simulink model "LowSpeed"  (R2022b)
settings: Solver=FixedStepDiscrete  StartTime=0.0  StopTime=10.0  FixedStep=0.0001  RelTol=1e-3
undefined symbols (not defined in the file or in its folder): DEPOWER_FLAG, DEPOWER_NO_FLAG, ParamCfg_IsMax_u16, ParamCfg_LowSpeedCoeff_u16, ParamCfg_LowSpeedDelay_u16, ParamCfg_LowSpeedGain_u16, ParamCfg_MaxTorque_u16, ParamCfg_SpeedLowLimit_u16
libraries: simulink x2
settings Model: DataDictionary=MCU_LowSpeed.sldd  Creator=ZYH  LastModifiedBy=ZYH
settings OptimizationCC: DefaultParameterBehavior=Inlined  EnhancedBackFolding=on  PassReuseOutputArgsAs=Individual arguments  ZeroExternalMemoryAtStartup=off  ZeroInternalMemoryAtStartup=off  OptimizeBlockOrder=speed  DifferentSizesBufferReuse=on  OptimizationCustomize=off  EfficientTunableParamExpr=on
settings DebuggingCC: ParameterTunabilityLossMsg=error
settings SFSimCC: MATLABDynamicMemAlloc=off
settings RTWCC: Description=Embedded Coder  SystemTargetFile=ert.tlc  GenCodeOnly=on  TemplateMakefile=ert_default_tmf
settings CodeAppCC: ForceParamTrailComments=on  IgnoreCustomStorageClasses=off  OperatorAnnotations=on  SimulinkDataObjDesc=on  SFDataObjDesc=on  InsertBlockDesc=on
settings ERTTargetCC: TargetLangStandard=C99 (ISO)  GenerateSampleERTMain=on  InlinedParameterPlacement=NonHierarchical  ERTCustomFileTemplate=example_file_process.tlc

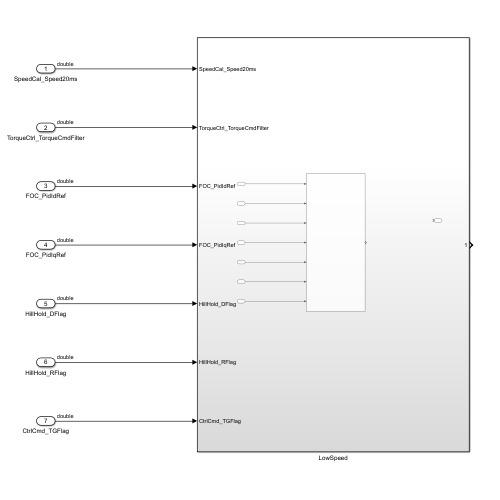
[thumbnail: Simulink's stored preview of the top-level diagram]
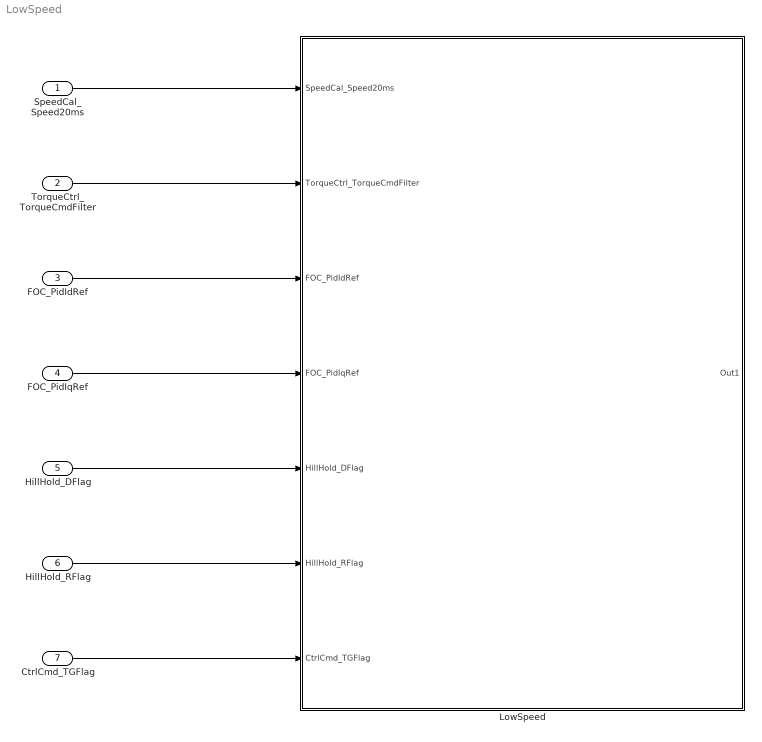
== system LowSpeed ==
  SpeedCal_Speed20ms : Inport
  TorqueCtrl_TorqueCmdFilter : Inport  Port=2
  FOC_PidIdRef : Inport  Port=3
  FOC_PidIqRef : Inport  Port=4
  HillHold_DFlag : Inport  Port=5
  HillHold_RFlag : Inport  Port=6
  CtrlCmd_TGFlag : Inport  Port=7
  LowSpeed : Subsystem
  wires:
  SpeedCal_Speed20ms/1 -> LowSpeed/1(SpeedCal_Speed20ms)
  TorqueCtrl_TorqueCmdFilter/1 -> LowSpeed/2(TorqueCtrl_TorqueCmdFilter)
  FOC_PidIdRef/1 -> LowSpeed/3(FOC_PidIdRef)
  FOC_PidIqRef/1 -> LowSpeed/4(FOC_PidIqRef)
  HillHold_DFlag/1 -> LowSpeed/5(HillHold_DFlag)
  HillHold_RFlag/1 -> LowSpeed/6(HillHold_RFlag)
  CtrlCmd_TGFlag/1 -> LowSpeed/7(CtrlCmd_TGFlag)

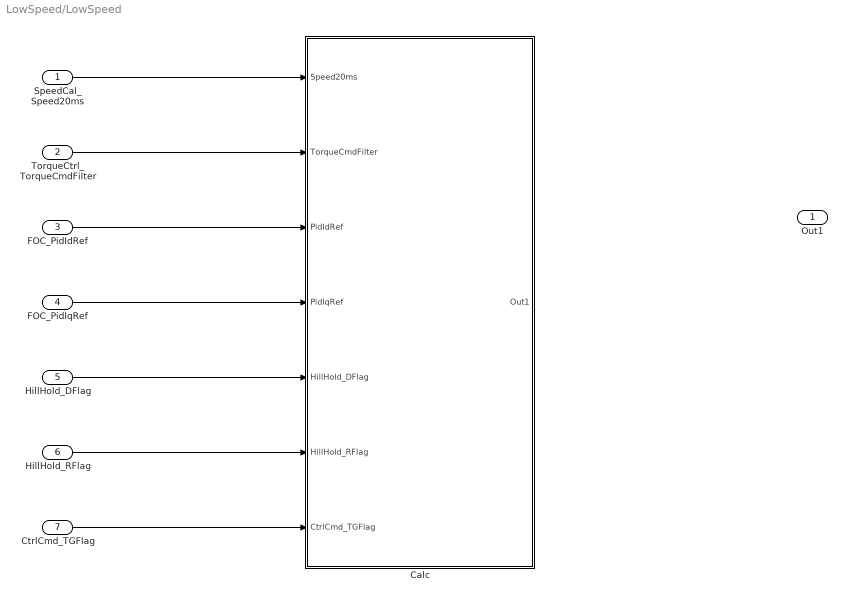
== system LowSpeed/LowSpeed ==
  SpeedCal_Speed20ms : Inport
  TorqueCtrl_TorqueCmdFilter : Inport  Port=2
  FOC_PidIdRef : Inport  Port=3
  FOC_PidIqRef : Inport  Port=4
  HillHold_DFlag : Inport  Port=5
  HillHold_RFlag : Inport  Port=6
  CtrlCmd_TGFlag : Inport  Port=7
  Calc : Subsystem
  Out1 : Outport
  wires:
  SpeedCal_Speed20ms/1 -> Calc/1(Speed20ms)
  TorqueCtrl_TorqueCmdFilter/1 -> Calc/2(TorqueCmdFilter)
  FOC_PidIdRef/1 -> Calc/3(PidIdRef)
  FOC_PidIqRef/1 -> Calc/4(PidIqRef)
  HillHold_DFlag/1 -> Calc/5(HillHold_DFlag)
  HillHold_RFlag/1 -> Calc/6(HillHold_RFlag)
  CtrlCmd_TGFlag/1 -> Calc/7(CtrlCmd_TGFlag)

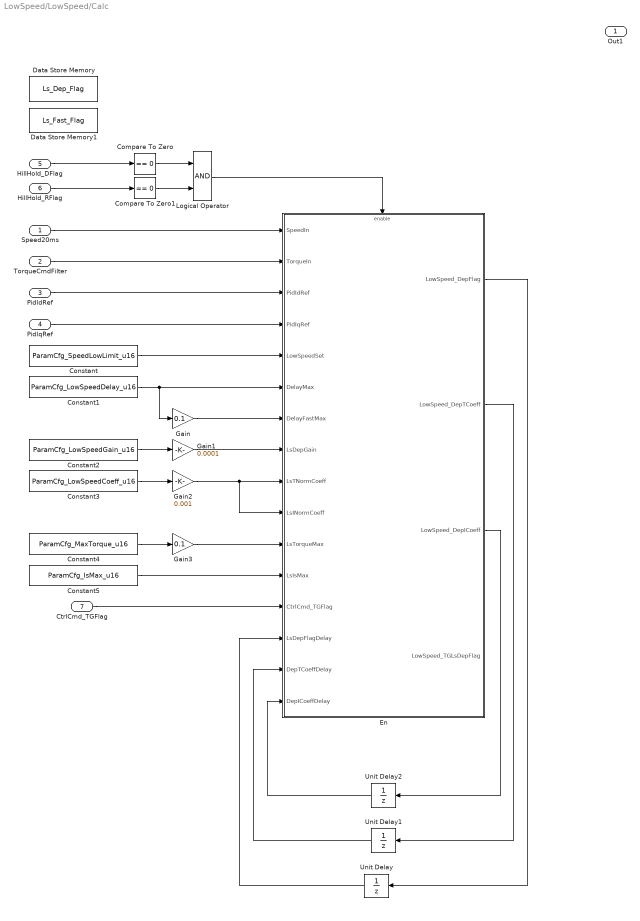
== system LowSpeed/LowSpeed/Calc ==
  Speed20ms : Inport
  TorqueCmdFilter : Inport  Port=2
  PidIdRef : Inport  Port=3
  PidIqRef : Inport  Port=4
  HillHold_DFlag : Inport  Port=5
  HillHold_RFlag : Inport  Port=6
  CtrlCmd_TGFlag : Inport  Port=7
  Compare To Zero : simulink/Logic and Bit Operations/Compare To Zero  relop===  OutDataTypeStr=boolean
  Compare To Zero1 : simulink/Logic and Bit Operations/Compare To Zero  relop===  OutDataTypeStr=boolean
  Constant : Constant  Value=ParamCfg_SpeedLowLimit_u16
  Constant1 : Constant  Value=ParamCfg_LowSpeedDelay_u16
  Constant2 : Constant  Value=ParamCfg_LowSpeedGain_u16
  Constant3 : Constant  Value=ParamCfg_LowSpeedCoeff_u16
  Constant4 : Constant  Value=ParamCfg_MaxTorque_u16
  Constant5 : Constant  Value=ParamCfg_IsMax_u16  VectorParams1D=off
  Data Store Memory : DataStoreMemory  DataStoreName=Ls_Dep_Flag  WriteAfterWriteMsg=warning  InitialValue=DEPOWER_NO_FLAG  ShowAdditionalParam=off  OutDataTypeStr=uint8
  Data Store Memory1 : DataStoreMemory  DataStoreName=Ls_Fast_Flag  WriteAfterWriteMsg=warning  InitialValue=false  ShowAdditionalParam=off  OutDataTypeStr=uint8
  En : Subsystem  TreatAsAtomicUnit=on
  Gain : Gain  Gain=0.1  ParamDataTypeStr=single  OutDataTypeStr=single
  Gain1 : Gain  Gain=0.0001  ParamDataTypeStr=single  OutDataTypeStr=single
  Gain2 : Gain  Gain=0.001  ParamDataTypeStr=single  OutDataTypeStr=single
  Gain3 : Gain  Gain=0.1  ParamDataTypeStr=single  OutDataTypeStr=single
  Logical Operator : Logic  AllPortsSameDT=off  OutDataTypeStr=boolean
  Unit Delay : UnitDelay  SampleTime=-1  HasFrameUpgradeWarning=on
  Unit Delay1 : UnitDelay  SampleTime=-1  HasFrameUpgradeWarning=on
  Unit Delay2 : UnitDelay  SampleTime=-1  HasFrameUpgradeWarning=on
  Out1 : Outport
  wires:
  HillHold_DFlag/1 -> Compare To Zero/1
  HillHold_RFlag/1 -> Compare To Zero1/1
  Compare To Zero1/1 -> Logical Operator/2
  Compare To Zero/1 -> Logical Operator/1
  Logical Operator/1 -> En/Enable
  Speed20ms/1 -> En/1(SpeedIn)
  TorqueCmdFilter/1 -> En/2(TorqueIn)
  PidIdRef/1 -> En/3(PidIdRef)
  PidIqRef/1 -> En/4(PidIqRef)
  Constant/1 -> En/5(LowSpeedSet)
  Gain/1 -> En/7(DelayFastMax)
  Constant1/1 -> Gain/1, En/6(DelayMax)
  Constant2/1 -> Gain1/1
  Gain1/1 -> En/8(LsDepGain)
  Constant3/1 -> Gain2/1
  Gain2/1 -> En/10(LsINormCoeff), En/9(LsTNormCoeff)
  Constant4/1 -> Gain3/1
  Gain3/1 -> En/11(LsTorqueMax)
  Constant5/1 -> En/12(LsIsMax)
  En/1(LowSpeed_DepFlag) -> Unit Delay/1
  Unit Delay/1 -> En/14(LsDepFlagDelay)
  En/2(LowSpeed_DepTCoeff) -> Unit Delay1/1
  Unit Delay1/1 -> En/15(DepTCoeffDelay)
  En/3(LowSpeed_DepICoeff) -> Unit Delay2/1
  Unit Delay2/1 -> En/16(DepICoeffDelay)
  CtrlCmd_TGFlag/1 -> En/13(CtrlCmd_TGFlag)

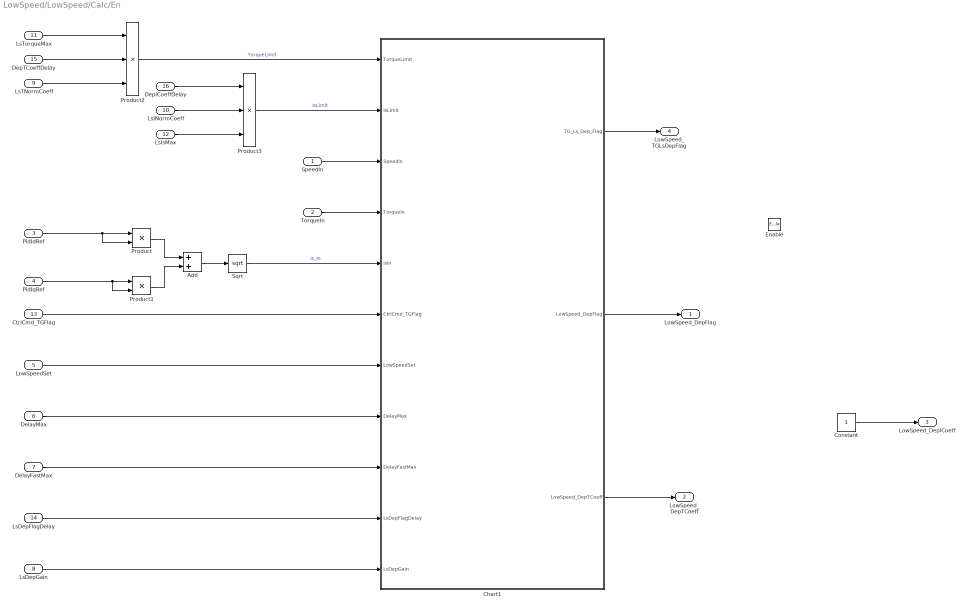
== system LowSpeed/LowSpeed/Calc/En ==
  SpeedIn : Inport
  TorqueIn : Inport  Port=2
  PidIdRef : Inport  Port=3
  PidIqRef : Inport  Port=4
  LowSpeedSet : Inport  Port=5
  DelayMax : Inport  Port=6
  DelayFastMax : Inport  Port=7
  LsDepGain : Inport  Port=8
  LsTNormCoeff : Inport  Port=9
  LsINormCoeff : Inport  Port=10
  LsTorqueMax : Inport  Port=11
  LsIsMax : Inport  Port=12
  CtrlCmd_TGFlag : Inport  Port=13
  LsDepFlagDelay : Inport  Port=14
  DepTCoeffDelay : Inport  Port=15
  DepICoeffDelay : Inport  Port=16
  Enable : EnablePort
  Add : Sum
  Chart1 : Stateflow chart  TreatAsAtomicUnit=on
  Constant : Constant  OutDataTypeStr=single
  Product : Product
  Product1 : Product
  Product2 : Product  Inputs=3
  Product3 : Product  Inputs=3
  Sqrt : Sqrt
  LowSpeed_DepFlag : Outport
  LowSpeed_DepTCoeff : Outport  Port=2
  LowSpeed_DepICoeff : Outport  Port=3
  LowSpeed_TGLsDepFlag : Outport  Port=4
  wires:
  PidIdRef/1 -> Product/2, Product/1
  PidIqRef/1 -> Product1/2, Product1/1
  Product/1 -> Add/1
  Product1/1 -> Add/2
  Add/1 -> Sqrt/1
  LsTorqueMax/1 -> Product2/1
  DepTCoeffDelay/1 -> Product2/2
  LsTNormCoeff/1 -> Product2/3
  LsINormCoeff/1 -> Product3/2
  DepICoeffDelay/1 -> Product3/1
  LsIsMax/1 -> Product3/3
  Product2/1 -> Chart1/1(TorqueLimit)  "TorqueLimit"
  Product3/1 -> Chart1/2(IsLimit)  "IsLimit"
  SpeedIn/1 -> Chart1/3(SpeedIn)
  TorqueIn/1 -> Chart1/4(TorqueIn)
  CtrlCmd_TGFlag/1 -> Chart1/6(CtrlCmd_TGFlag)
  Sqrt/1 -> Chart1/5(IsIn)  "Is_In"
  LowSpeedSet/1 -> Chart1/7(LowSpeedSet)
  DelayMax/1 -> Chart1/8(DelayMax)
  DelayFastMax/1 -> Chart1/9(DelayFastMax)
  LsDepFlagDelay/1 -> Chart1/10(LsDepFlagDelay)
  LsDepGain/1 -> Chart1/11(LsDepGain)
  Chart1/2(LowSpeed_DepFlag) -> LowSpeed_DepFlag/1
  Chart1/1(TG_Ls_Dep_Flag) -> LowSpeed_TGLsDepFlag/1
  Chart1/3(LowSpeed_DepTCoeff) -> LowSpeed_DepTCoeff/1
  Constant/1 -> LowSpeed_DepICoeff/1

== stateflow chart LowSpeed/Calc/En/Chart1 ==
  (default) -> (junction 1) : {Ls_Dep_Flag = LsDepFlagDelay;}
  (junction 1) -> (junction 7) [order 1] : [abs(SpeedIn)<LowSpeedSet && (abs(TorqueIn)>TorqueLimit ||IsIn>IsLimit)]
  (junction 1) -> (junction 11) [order 2]
  (junction 7) -> (junction 9) : {
      | DelayCnt = DelayCnt+1;
      | FastCnt = FastCnt + 1;
      | }
  (junction 9) -> (junction 24) : [DelayCnt>DelayMax]
  (junction 24) -> (junction 28)
  (junction 28) -> (junction 30) [order 1] : [TorqueLimit > 0.001 || IsLimit>0.001]
  (junction 28) -> (junction 36) [order 2] : {DelayCnt = DelayCnt-1}
  (junction 30) -> (junction 32) : {Ls_Dep_Flag = DEPOWER_FLAG}
  (junction 11) -> (junction 13) [order 1] : [CtrlCmd_TGFlag == 0]
  (junction 11) -> (junction 51) [order 2]
  (junction 13) -> (junction 16)
  (junction 32) -> (junction 36)
  (junction 36) -> (junction 39)
  (junction 16) -> (junction 18) [order 1] : [Ls_Dep_Flag == DEPOWER_FLAG]
  (junction 16) -> (junction 55) [order 2] : {TG_Ls_Dep_Flag =false}
  (junction 18) -> (junction 53) : {TG_Ls_Dep_Flag =true}
  (junction 39) -> (junction 41) [order 1] : [FastCnt > DelayFastMax]
  (junction 39) -> (junction 45) [order 2]
  (junction 41) -> (junction 43) : {
      | Ls_Fast_Flag = DEPOWER_FLAG;
      | FastCnt = DelayFastMax
      | }
  (junction 53) -> (junction 55)
  (junction 55) -> (junction 58) : {
      | DelayCnt = 0;
      | FastCnt =0;
      | Ls_Dep_Flag = DEPOWER_NO_FLAG;
      | Ls_Fast_Flag = DEPOWER_NO_FLAG;
      | }
  (junction 43) -> (junction 45)
  (junction 45) -> (junction 49)
  (junction 58) -> (junction 51)
  (junction 51) -> (junction 63)
  (junction 49) -> (junction 63)
  (junction 63) -> (junction 66)
  (junction 66) -> (junction 69) [order 1] : [Ls_Dep_Flag ==DEPOWER_FLAG ]
  (junction 66) -> (junction 71) [order 2] : {Ls_Dep_Coeff = 1}
  (junction 69) -> (junction 73) : {Ls_Dep_Coeff = 1-LsDepGain*(DelayCnt-FastCnt)}
  (junction 73) -> (junction 75) [order 1] : [Ls_Dep_Coeff < 0.001]
      | {Ls_Dep_Coeff = 0}
  (junction 73) -> (junction 75) [order 2]
  (junction 75) -> (junction 79) [order 2]
  (junction 75) -> (junction 79) [order 1] : [Ls_Dep_Coeff > 1]
      | {Ls_Dep_Coeff = 1}
  (junction 79) -> (junction 71)
  (junction 71) -> (junction 86) : {
      | LowSpeed_DepTCoeff = Ls_Dep_Coeff;
      | LowSpeed_DepFlag = Ls_Dep_Flag;
      |
      | }
  data: TorqueLimit input; IsLimit input; SpeedIn input; TorqueIn input; IsIn input; CtrlCmd_TGFlag input; LowSpeedSet input; DelayCnt local uint16 =0; FastCnt local uint16 =0; DelayMax input; DelayFastMax input; DEPOWER_FLAG parameter; Ls_Dep_Flag data_store_memory; Ls_Fast_Flag data_store_memory; TG_Ls_Dep_Flag output uint8 =0; LowSpeed_DepFlag output uint8 =0; DEPOWER_NO_FLAG parameter; LsDepFlagDelay input; LsDepGain input; Ls_Dep_Coeff local single; LowSpeed_DepTCoeff output single
